simulink model "new_inkine_2020"  (R2022b)
settings: Solver=FixedStepAuto  StartTime=0.0  StopTime=250  FixedStep=0.001  RelTol=1e-3
PreLoadFcn:
  | parameters_new;
InitFcn:
  | parameters_new;
(part 3 of 3)

== matlab function new_inkine_2020/Subsystem/MATLAB Function1 ==
  data: tau0 output; a input; tau output; q input; dq input; d2q input; Wn input; Z2 input; adaptive_rate output
function [tau0,tau,adaptive_rate] = fcn(a,q,dq,d2q, Wn,Z2)
% S1,L1,L3,M1,M2,R2,R1,Le,K1,...
% L2,L11,S3,S4,Lc14,Lc14y,LC1,LC1y,LC2,LC2y,LC3,...
% L9,Lcx10,Ls5,Ls6,Ls11,Ls13,... %杆长与偏置
% I1,I2,I3,I4,I5,I6,I7,I8,I9,I10,I11,I12,I13,I14,I15,...
g=9806.65;theta6=5*pi/6; theta7=-pi/6;
coder.extrinsic('evalin');
L1=0;L3=0;S1=0;R1=0;R2=0;Le=0;K1=0;K2=0;M1=0;M2=0;
L1=evalin('base','L1');L3=evalin('base','L3');S1=evalin('base','S1');R1=evalin('base','R1');Le=evalin('base','Le');R2=evalin('base','R2');
K1=evalin('base','K1');K2=evalin('base','K2');M1=evalin('base','M1');M2=evalin('base','M2');
S1=82;L1=600;L3=550;M1=312.5;M2=140.5;R2=318;
R1=200;Le=414;K1=270;L2=215;L11=532;S3=150;S4=180;
Lc14=100.63;Lc14y=49.13;LC1=192.36;
LC1y=7.69;LC2=-38.71;LC2y=-48.68;LC3=167.99;
L9=sqrt(4.13^2+2.45^2);Lcx10=-13.9;
Ls5=268.5;Ls6=-242.5;Ls11=189; Ls13=189; %偏置

% m1=31.235;m2=17.983;m3=21.85;m4=5.16;m5=2.248;m6=2.248;m7=1.73;m8=1.73;
% m9=121.413;m10=13.425;m11=3.54;m12=1.729;m13=2.99;m14=5.342;m15=2.79;
% I1=[531432.895,1962865.034,1545286.115];
% I2=[118284.16,456199.27,500258.95];
% I3=[79013.25, 1135425.11, 1121439.73];
% I4=[870.60,179377.20,179369.49];
% I5=[3169.766,5265.289,3886.288];%滑块1
% I6=[3169.766,5265.289,3886.288];%滑块2
% I7=[143.00,29009.62,29008.38];
% I8=[143.00,29009.62,29008.38];%AC,BC
% I9=[5187204.097,6638143.629, 4645540.195];
% I10=[230616.784, 122346.017, 246696.850];
% I11=[10700.52,125437.80,115850.13];
% I12=[12209.748,498.623,12408.157];
% I13=[397.49,124363.03,124495.89];
% I14=[18845.358,28753.446,45020.107];
% I15=[376.19,99421.54,99541.62];

m1=51.81;m2=19.166;m3=39.652;m4=8.609;m5=2.248;m6=2.248;m7=3.094;m8=3.094;m9=121.413;m10=11.03; 
m11=8.433;m12=2.164;m13=3.27;m14=5.342;m15=3.585;
I1=[799946.49,3888376.65,3292839.24];
I2=[141847.10, 540821.180,573215.730];
I3=[184132.217, 2737294.136, 2737294.136];
I4=[3478.492,396735.669,396757.714];
I5=[3169.766,5265.289,3886.288];
I6=[3169.766,5265.289,3886.288];
I7=[1032.344, 86107.112,86524.495];
I8=[1032.344, 86107.112,86524.495];
I9=[5187204.097,6638143.629, 4645540.195];
I10=[ 96918.57, 207811.09,  196352.11];
I11=[19267.104,306573.070,298677.886];
I12=[12641.763,1276.684,12641.763];
I13=[1031.019,155951.918, 156712.730];
I14=[18845.358,28753.446,45020.107];
I15=[1180.720,164711.775,165542.954];

K2=K1;L7=Le;L8=L7;Lc11=45+0.5*L11;Lc13=0.5*L1;Lc15=0.5*L3;
% m1=m(1);m2=m(2);m3=m(3);m4=m(4);m5=m(5);m6=m(6);m7=m(7);m8=m(8);m9=m(9);m10=m(10);m11=m(11);m12=m(12);m13=m(13);m14=m(14);m15=m(15);

mload=50;

Ixx1=I1(1); Iyy1=I1(2); Izz1=I1(3);
Ixx2=I2(1); Iyy2=I2(2); Izz2=I2(3);
Ixx3=I3(1); Iyy3=I3(2); Izz3=I3(3);
Ixx4=I4(1); Iyy4=I4(2); Izz4=I4(3);
Ixx5=I5(1); Iyy5=I5(2); Izz5=I5(3);
Ixx6=I6(1); Iyy6=I6(2); Izz6=I6(3);
Ixx7=I7(1); Iyy7=I7(2); Izz7=I7(3);
Ixx8=I8(1); Iyy8=I8(2); Izz8=I8(3);
Ixx9=I9(1); Iyy9=I9(2); Izz9=I9(3);
Ixx10=I10(1);Iyy10=I10(2);Izz10=I10(3);
Ixx11=I11(1);Iyy11=I11(2);Izz11=I11(3);
Ixx12=I12(1);Iyy12=I12(2);Izz12=I12(3);
Ixx13=I13(1);Iyy13=I13(2);Izz13=I13(3);
Ixx14=I14(1);Iyy14=I14(2);Izz14=I14(3);
Ixx15=I15(1);Iyy15=I15(2);Izz15=I15(3);



theta1=q(1);theta4=q(2);theta5=q(3);
theta2=theta6-theta4;theta3=theta7-theta5;
dq1=dq(1);dq2=dq(2);dq3=dq(3);

n=sqrt((M1 - R2*cos(theta3))^2 + (M2 - R2*sin(theta3))^2);n1=1/n;
phi1=asin((K1-R1*sin(theta2))/L7);
phi2=acos((K2-R1*cos(theta2))/L8);
cph1=(L7^2-(K1-R1*sin(theta2))^2)^0.5/L7;

jij9=[ Izz9, 0, 0;0,0,0;0,0,0];Ekr9=0.5*dq.'*jij9*dq;
jmj9=[ L9^2*m9, 0, 0; 0, 0, 0;0, 0, 0];Ekt9=0.5*dq.'*jmj9*dq;

Mm=[Ixx5 + Iyy14/2 + Izz6 + Izz9 + Izz10 + (2*Lc11*m11*sin(theta1)*(M1 - R2*cos(theta5 - theta7))*(Ls11*cos(theta1) - sin(theta1)*(M1 - S1)) - 2*Lc11*m11*cos(theta1)*(M1 - R2*cos(theta5 - theta7))*(Ls11*sin(theta1) + cos(theta1)*(M1 - S1)))*n1 + (Lc11^2*m11*cos(theta1)^2*(M1 - R2*cos(theta5 - theta7))^2 + Lc11^2*m11*sin(theta1)^2*(M1 - R2*cos(theta5 - theta7))^2)*n1^2 + Ixx14/2 - Ixx8*((K2 - R1*cos(theta4 - theta6))^2/L8^2 - 1) + Iyy1*cos(theta4)^2 + Iyy2*cos(theta5)^2 + Iyy3*cos(theta5)^2 + Iyy4*cos(theta4)^2 + Iyy13*cos(theta4)^2 + Iyy15*cos(theta5)^2 - Iyy7*((K1 + R1*sin(theta4 - theta6))^2/L7^2 - 1) + Ixx1*sin(theta4)^2 + Ixx2*sin(theta5)^2 + Ixx3*sin(theta5)^2 + Ixx4*sin(theta4)^2 + Ixx13*sin(theta4)^2 + Ixx15*sin(theta5)^2 + (Iyy8*(K2 - R1*cos(theta4 - theta6))^2)/L8^2 + (Ixx7*(K1 + R1*sin(theta4 - theta6))^2)/L7^2 + Iyy11*n1^2*(M1 - R2*cos(theta5 - theta7))^2 + Ixx11*n1^2*(M2 + R2*sin(theta5 - theta7))^2 + (Ixx12*(M1 - R2*cos(theta5 - theta7))^2)/((M1 - R2*cos(theta5 - theta7))^2 + (M2 + R2*sin(theta5 - theta7))^2) + (Izz12*(M2 + R2*sin(theta5 - theta7))^2)/((M1 - R2*cos(theta5 - theta7))^2 + (M2 + R2*sin(theta5 - theta7))^2) + (m13*(4*Lc13^2*cos(theta4)^2 - 8*Lc13*S1*cos(theta4) - 4*sqrt((3))*Lc13*S3*cos(theta4) + 4*Ls13^2 + 4*S1^2 + 4*sqrt((3))*S1*S3 + 3*S3^2))/4 + m15*(sin(theta1)*(S1 + (sqrt((2))*S4)/2 - L1*cos(theta4) - Lc15*cos(theta5)) + Ls13*cos(theta1))^2 + m15*(cos(theta1)*(S1 + (sqrt((2))*S4)/2 - L1*cos(theta4) - Lc15*cos(theta5)) - Ls13*sin(theta1))^2 + m6*(K2^2 - 2*K2*S1 + Ls6^2 + S1^2) + (m4*(2*S1 - L1*cos(theta4) + 2*L2*cos(theta5))^2)/4 + m3*(L1*cos(theta4) - S1 + LC3*cos(theta5))^2 + m1*(LC1*cos(theta4) - S1 + LC1y*sin(theta4))^2 + (m14*(cos(theta1)*(Lc14y + 2*S1 - sqrt((3))*Lc14 + sqrt((3))*S3 - 2*L1*cos(theta4)) - 2*Ls13*sin(theta1))^2)/4 + (m14*(sin(theta1)*(Lc14y + 2*S1 - sqrt((3))*Lc14 + sqrt((3))*S3 - 2*L1*cos(theta4)) + 2*Ls13*cos(theta1))^2)/4 + m10*(Lcx10 - S1 + L1*cos(theta4) + L3*cos(theta5))^2 + m5*(sin(theta1)*(S1 + sqrt(L7^2 - (K1 + R1*sin(theta4 - theta6))^2) - R1*cos(theta4 - theta6)) + Ls5*cos(theta1))^2 + m5*(cos(theta1)*(S1 + sqrt(L7^2 - (K1 + R1*sin(theta4 - theta6))^2) - R1*cos(theta4 - theta6)) - Ls5*sin(theta1))^2 + (m7*(L7^2*cph1^2 - 4*L7*R1*cph1*cos(theta4 - theta6) + 4*L7*S1*cph1 + 4*Ls5^2 + 4*R1^2*cos(theta4 - theta6)^2 - 8*R1*S1*cos(theta4 - theta6) + 4*S1^2))/4 + L9^2*m9 + (m8*(K2^2 + 2*K2*R1*cos(theta4 - theta6) - 4*K2*S1 + 4*Ls6^2 + R1^2*cos(theta4 - theta6)^2 - 4*R1*S1*cos(theta4 - theta6) + 4*S1^2))/4 + m12*(S1 - R2*cos(theta5 - theta7))^2 + m11*(Ls11*sin(theta1) + cos(theta1)*(M1 - S1))^2 + m11*(Ls11*cos(theta1) - sin(theta1)*(M1 - S1))^2 + m2*(S1 + LC2*cos(theta5) - LC2y*sin(theta5))^2, - L1*Ls13*m14*sin(theta4) - L1*Ls13*m15*sin(theta4) - Lc13*Ls13*m13*sin(theta4) - (Ls6*R1*m8*sin(theta4 - theta6))/2 + (Ls5*R1*m5*((R1*sin(2*theta4 - 2*theta6))/2 - sin(theta4 - theta6)*sqrt(L7^2 - (K1 + R1*sin(theta4 - theta6))^2) + K1*cos(theta4 - theta6)))/sqrt(L7^2 - (K1 + R1*sin(theta4 - theta6))^2) + (Ls5*R1*m7*(K1*cos(theta4 - theta6) - 2*L7*cph1*sin(theta4 - theta6) + R1*cos(theta4 - theta6)*sin(theta4 - theta6)))/(2*L7*cph1), (-Lc11*Ls11*R2*m11*(M2 + R2*sin(theta5 - theta7))*(R2 - M1*cos(theta5 - theta7) + M2*sin(theta5 - theta7)))*n1^3 - Lc15*Ls13*m15*sin(theta5); - L1*Ls13*m14*sin(theta4) - L1*Ls13*m15*sin(theta4) - Lc13*Ls13*m13*sin(theta4) - (Ls6*R1*m8*sin(theta4 - theta6))/2 + (Ls5*R1*m5*((R1*sin(2*theta4 - 2*theta6))/2 - sin(theta4 - theta6)*sqrt(L7^2 - (K1 + R1*sin(theta4 - theta6))^2) + K1*cos(theta4 - theta6)))/sqrt(L7^2 - (K1 + R1*sin(theta4 - theta6))^2) + (Ls5*R1*m7*(K1*cos(theta4 - theta6) - 2*L7*cph1*sin(theta4 - theta6) + R1*cos(theta4 - theta6)*sin(theta4 - theta6)))/(2*L7*cph1), Izz1 + Izz4 + Izz13 + m6*(R1*cos(theta4 - theta6) - (R1*sin(theta4 - theta6)*(K2 - R1*cos(theta4 - theta6)))/sqrt(L7^2 - (K2 - R1*cos(theta4 - theta6))^2))^2 + L1^2*m10 + L1^2*m3 + (L1^2*m4)/4 + L1^2*m14 + L1^2*m15 + Lc13^2*m13 + m1*(LC1^2 + LC1y^2) + m8*(R1*cos(theta4 - theta6) - (R1*sin(theta4 - theta6)*(K2 - R1*cos(theta4 - theta6)))/(L8*sqrt(1 - (K2 - R1*cos(theta4 - theta6))^2/L8^2)*2))^2 + m7*cos(theta1)^2*(R1*sin(theta4 - theta6) - (R1*cos(theta4 - theta6)*(K1 + R1*sin(theta4 - theta6)))/(2*L7*cph1))^2 + m7*sin(theta1)^2*(R1*sin(theta4 - theta6) - (R1*cos(theta4 - theta6)*(K1 + R1*sin(theta4 - theta6)))/(2*L7*cph1))^2 + m5*cos(theta1)^2*(R1*sin(theta4 - theta6) - (R1*cos(theta4 - theta6)*(K1 + R1*sin(theta4 - theta6)))/sqrt(L7^2 - (K1 + R1*sin(theta4 - theta6))^2))^2 + m5*sin(theta1)^2*(R1*sin(theta4 - theta6) - (R1*cos(theta4 - theta6)*(K1 + R1*sin(theta4 - theta6)))/sqrt(L7^2 - (K1 + R1*sin(theta4 - theta6))^2))^2 + (R1^2*m7*cos(theta4 - theta6)^2)/4 + (R1^2*m8*sin(theta4 - theta6)^2*cos(theta1)^2)/4 + (R1^2*m8*sin(theta4 - theta6)^2*sin(theta1)^2)/4 - (Izz7*R1^2*cos(theta4 - theta6)^2)/(L7^2*((K1 + R1*sin(theta4 - theta6))^2/L7^2 - 1)) - (Izz8*R1^2*sin(theta4 - theta6)^2)/(L8^2*((K2 - R1*cos(theta4 - theta6))^2/L8^2 - 1)), L1*L3*cos(theta4 - theta5)*m10 - (L1*L2*m4*cos(theta4 - theta5))/2 + L1*LC3*m3*cos(theta4 - theta5) + L1*Lc15*m15*cos(theta4 - theta5); (-Lc11*Ls11*R2*m11*(M2 + R2*sin(theta5 - theta7))*(R2 - M1*cos(theta5 - theta7) + M2*sin(theta5 - theta7)))*n1^3 - Lc15*Ls13*m15*sin(theta5), L1*L3*cos(theta4 - theta5)*m10 - (L1*L2*m4*cos(theta4 - theta5))/2 + L1*LC3*m3*cos(theta4 - theta5) + L1*Lc15*m15*cos(theta4 - theta5), Izz2 + Izz3 + Izz15 + (Lc11^2*R2^2*m11*(M1 - R2*cos(theta5 - theta7))^2*(R2 - M1*cos(theta5 - theta7) + M2*sin(theta5 - theta7))^2 + Lc11^2*R2^2*m11*cos(theta1)^2*(M2 + R2*sin(theta5 - theta7))^2*(R2 - M1*cos(theta5 - theta7) + M2*sin(theta5 - theta7))^2 + Lc11^2*R2^2*m11*sin(theta1)^2*(M2 + R2*sin(theta5 - theta7))^2*(R2 - M1*cos(theta5 - theta7) + M2*sin(theta5 - theta7))^2)*n1^6 - (Iyy12*((R2*sin(theta5 - theta7))/sqrt(((M1 - R2*cos(theta5 - theta7))^2 + (M2 + R2*sin(theta5 - theta7))^2)) - ((M1 - R2*cos(theta5 - theta7))*(2*R2*cos(theta5 - theta7)*(M2 + R2*sin(theta5 - theta7)) + 2*R2*sin(theta5 - theta7)*(M1 - R2*cos(theta5 - theta7))))/(2*((M1 - R2*cos(theta5 - theta7))^2 + (M2 + R2*sin(theta5 - theta7))^2)^(3/2)))^2)/((M1 - R2*cos(theta5 - theta7))^2/((M1 - R2*cos(theta5 - theta7))^2 + (M2 + R2*sin(theta5 - theta7))^2) - 1) + Izz11*R2^2*n1^4*(R2 - M1*cos(theta5 - theta7) + M2*sin(theta5 - theta7))^2 + m4*L2^2 + m10*L3^2 + m3*LC3^2 + m15*Lc15^2 + m12*R2^2 + m2*(LC2^2 + LC2y^2)];

V2=[dq1*((dq3*(2*R2*m11*sin(theta5 - theta7)*(M1 - R2*cos(theta5 - theta7))*Lc11^2*cos(theta1)^2 + 2*R2*m11*sin(theta5 - theta7)*(M1 - R2*cos(theta5 - theta7))*Lc11^2*sin(theta1)^2)*n1^2)/2 - (dq3*(2*Lc11*R2*m11*sin(theta5 - theta7)*cos(theta1)*(Ls11*sin(theta1) + cos(theta1)*(M1 - S1)) - 2*Lc11*R2*m11*sin(theta5 - theta7)*sin(theta1)*(Ls11*cos(theta1) - sin(theta1)*(M1 - S1)))*n1)/2 + (dq2*((m13*(8*Lc13*S1*sin(theta4) - 8*Lc13^2*cos(theta4)*sin(theta4) + 4*sqrt((3))*Lc13*S3*sin(theta4)))/4 - (m8*(2*K2*R1*sin(theta4 - theta6) - 4*R1*S1*sin(theta4 - theta6) + 2*R1^2*cos(theta4 - theta6)*sin(theta4 - theta6)))/4 + (m7*(8*R1*S1*sin(theta4 - theta6) - 8*R1^2*cos(theta4 - theta6)*sin(theta4 - theta6) + 4*L7*R1*cph1*sin(theta4 - theta6)))/4 + 2*Ixx1*cos(theta4)*sin(theta4) + 2*Ixx4*cos(theta4)*sin(theta4) + 2*Ixx13*cos(theta4)*sin(theta4) - 2*Iyy1*cos(theta4)*sin(theta4) - 2*Iyy4*cos(theta4)*sin(theta4) - 2*Iyy13*cos(theta4)*sin(theta4) + 2*m1*(LC1y*cos(theta4) - LC1*sin(theta4))*(LC1*cos(theta4) - S1 + LC1y*sin(theta4)) + (L1*m4*sin(theta4)*(2*S1 - L1*cos(theta4) + 2*L2*cos(theta5)))/2 - 2*L1*m3*sin(theta4)*(L1*cos(theta4) - S1 + LC3*cos(theta5)) - 2*L1*sin(theta4)*m10*(Lcx10 - S1 + L1*cos(theta4) + L3*cos(theta5)) + 2*m5*cos(theta1)*(cos(theta1)*(S1 + sqrt((L7^2 - (K1 + R1*sin(theta4 - theta6))^2)) - R1*cos(theta4 - theta6)) - Ls5*sin(theta1))*(R1*sin(theta4 - theta6) - (R1*cos(theta4 - theta6)*(K1 + R1*sin(theta4 - theta6)))/sqrt(L7^2 - (K1 + R1*sin(theta4 - theta6))^2)) + 2*m5*sin(theta1)*(sin(theta1)*(S1 + sqrt((L7^2 - (K1 + R1*sin(theta4 - theta6))^2)) - R1*cos(theta4 - theta6)) + Ls5*cos(theta1))*(R1*sin(theta4 - theta6) - (R1*cos(theta4 - theta6)*(K1 + R1*sin(theta4 - theta6)))/sqrt(L7^2 - (K1 + R1*sin(theta4 - theta6))^2)) + L1*m14*cos(theta1)*sin(theta4)*(cos(theta1)*(Lc14y + 2*S1 - sqrt((3))*Lc14 + sqrt((3))*S3 - 2*L1*cos(theta4)) - 2*Ls13*sin(theta1)) + L1*m14*sin(theta1)*sin(theta4)*(sin(theta1)*(Lc14y + 2*S1 - sqrt((3))*Lc14 + sqrt((3))*S3 - 2*L1*cos(theta4)) + 2*Ls13*cos(theta1)) + (2*Ixx7*R1*cos(theta4 - theta6)*(K1 + R1*sin(theta4 - theta6)))/L7^2 - (2*Ixx8*R1*sin(theta4 - theta6)*(K2 - R1*cos(theta4 - theta6)))/L8^2 - (2*Iyy7*R1*cos(theta4 - theta6)*(K1 + R1*sin(theta4 - theta6)))/L7^2 + (2*Iyy8*R1*sin(theta4 - theta6)*(K2 - R1*cos(theta4 - theta6)))/L8^2 + 2*L1*m15*cos(theta1)*sin(theta4)*(cos(theta1)*(S1 + (sqrt((2))*S4)/2 - L1*cos(theta4) - Lc15*cos(theta5)) - Ls13*sin(theta1)) + 2*L1*m15*sin(theta1)*sin(theta4)*(sin(theta1)*(S1 + (sqrt((2))*S4)/2 - L1*cos(theta4) - Lc15*cos(theta5)) + Ls13*cos(theta1))))/2 + (dq3*(2*Ixx2*cos(theta5)*sin(theta5) - 2*m2*(LC2y*cos(theta5) + LC2*sin(theta5))*(S1 + LC2*cos(theta5) - LC2y*sin(theta5)) + 2*Ixx3*cos(theta5)*sin(theta5) + 2*Ixx15*cos(theta5)*sin(theta5) - 2*Iyy2*cos(theta5)*sin(theta5) - 2*Iyy3*cos(theta5)*sin(theta5) - 2*Iyy15*cos(theta5)*sin(theta5) - L2*m4*sin(theta5)*(2*S1 - L1*cos(theta4) + 2*L2*cos(theta5)) - 2*LC3*m3*sin(theta5)*(L1*cos(theta4) - S1 + LC3*cos(theta5)) - 2*L3*sin(theta5)*m10*(Lcx10 - S1 + L1*cos(theta4) + L3*cos(theta5)) - (Ixx12*(M1 - R2*cos(theta5 - theta7))^2*(2*R2*cos(theta5 - theta7)*(M2 + R2*sin(theta5 - theta7)) + 2*R2*sin(theta5 - theta7)*(M1 - R2*cos(theta5 - theta7))))/((M1 - R2*cos(theta5 - theta7))^2 + (M2 + R2*sin(theta5 - theta7))^2)^2 + 2*R2*m12*sin(theta5 - theta7)*(S1 - R2*cos(theta5 - theta7)) - (Izz12*(M2 + R2*sin(theta5 - theta7))^2*(2*R2*cos(theta5 - theta7)*(M2 + R2*sin(theta5 - theta7)) + 2*R2*sin(theta5 - theta7)*(M1 - R2*cos(theta5 - theta7))))/((M1 - R2*cos(theta5 - theta7))^2 + (M2 + R2*sin(theta5 - theta7))^2)^2 + 2*Ixx11*R2*n1^2*cos(theta5 - theta7)*(M2 + R2*sin(theta5 - theta7)) + 2*Iyy11*R2*n1^2*sin(theta5 - theta7)*(M1 - R2*cos(theta5 - theta7)) + 2*Lc15*m15*cos(theta1)*sin(theta5)*(cos(theta1)*(S1 + (sqrt((2))*S4)/2 - L1*cos(theta4) - Lc15*cos(theta5)) - Ls13*sin(theta1)) + 2*Lc15*m15*sin(theta1)*sin(theta5)*(sin(theta1)*(S1 + (sqrt((2))*S4)/2 - L1*cos(theta4) - Lc15*cos(theta5)) + Ls13*cos(theta1)) + (2*Ixx12*R2*sin(theta5 - theta7)*(M1 - R2*cos(theta5 - theta7)))/((M1 - R2*cos(theta5 - theta7))^2 + (M2 + R2*sin(theta5 - theta7))^2) + (2*Izz12*R2*cos(theta5 - theta7)*(M2 + R2*sin(theta5 - theta7)))/((M1 - R2*cos(theta5 - theta7))^2 + (M2 + R2*sin(theta5 - theta7))^2)))/2) - dq2*(dq2*(L1*Ls13*m14*cos(theta4) + L1*Ls13*m15*cos(theta4) + Lc13*Ls13*m13*cos(theta4) + (Ls6*R1*m8*cos(theta4 - theta6))/2 + (Ls5*R1*m5*(cos(theta4 - theta6)*sqrt((L7^2 - (K1 + R1*sin(theta4 - theta6))^2)) - R1*cos(2*theta4 - 2*theta6) + K1*sin(theta4 - theta6) - (R1*cos(theta4 - theta6)*sin(theta4 - theta6)*(K1 + R1*sin(theta4 - theta6)))/sqrt((L7^2 - (K1 + R1*sin(theta4 - theta6))^2))))/sqrt((L7^2 - (K1 + R1*sin(theta4 - theta6))^2)) + (Ls5*R1*m7*(- R1*cos(theta4 - theta6)^2 + 2*L7*cph1*cos(theta4 - theta6) + R1*sin(theta4 - theta6)^2 + K1*sin(theta4 - theta6)))/(2*L7*cph1) - (Ls5*R1^2*m5*cos(theta4 - theta6)*(K1 + R1*sin(theta4 - theta6))*((R1*sin(2*theta4 - 2*theta6))/2 - sin(theta4 - theta6)*sqrt((L7^2 - (K1 + R1*sin(theta4 - theta6))^2)) + K1*cos(theta4 - theta6)))/(L7^2 - (K1 + R1*sin(theta4 - theta6))^2)^(3/2)) - (dq1*((m13*(8*Lc13*S1*sin(theta4) - 8*Lc13^2*cos(theta4)*sin(theta4) + 4*sqrt((3))*Lc13*S3*sin(theta4)))/4 - (m8*(2*K2*R1*sin(theta4 - theta6) - 4*R1*S1*sin(theta4 - theta6) + 2*R1^2*cos(theta4 - theta6)*sin(theta4 - theta6)))/4 + (m7*(8*R1*S1*sin(theta4 - theta6) - 8*R1^2*cos(theta4 - theta6)*sin(theta4 - theta6) + 4*L7*R1*cph1*sin(theta4 - theta6)))/4 + 2*Ixx1*cos(theta4)*sin(theta4) + 2*Ixx4*cos(theta4)*sin(theta4) + 2*Ixx13*cos(theta4)*sin(theta4) - 2*Iyy1*cos(theta4)*sin(theta4) - 2*Iyy4*cos(theta4)*sin(theta4) - 2*Iyy13*cos(theta4)*sin(theta4) + 2*m1*(LC1y*cos(theta4) - LC1*sin(theta4))*(LC1*cos(theta4) - S1 + LC1y*sin(theta4)) + (L1*m4*sin(theta4)*(2*S1 - L1*cos(theta4) + 2*L2*cos(theta5)))/2 - 2*L1*m3*sin(theta4)*(L1*cos(theta4) - S1 + LC3*cos(theta5)) - 2*L1*sin(theta4)*m10*(Lcx10 - S1 + L1*cos(theta4) + L3*cos(theta5)) + 2*m5*cos(theta1)*(cos(theta1)*(S1 + sqrt((L7^2 - (K1 + R1*sin(theta4 - theta6))^2)) - R1*cos(theta4 - theta6)) - Ls5*sin(theta1))*(R1*sin(theta4 - theta6) - (R1*cos(theta4 - theta6)*(K1 + R1*sin(theta4 - theta6)))/sqrt(L7^2 - (K1 + R1*sin(theta4 - theta6))^2)) + 2*m5*sin(theta1)*(sin(theta1)*(S1 + sqrt((L7^2 - (K1 + R1*sin(theta4 - theta6))^2)) - R1*cos(theta4 - theta6)) + Ls5*cos(theta1))*(R1*sin(theta4 - theta6) - (R1*cos(theta4 - theta6)*(K1 + R1*sin(theta4 - theta6)))/sqrt(L7^2 - (K1 + R1*sin(theta4 - theta6))^2)) + L1*m14*cos(theta1)*sin(theta4)*(cos(theta1)*(Lc14y + 2*S1 - sqrt((3))*Lc14 + sqrt((3))*S3 - 2*L1*cos(theta4)) - 2*Ls13*sin(theta1)) + L1*m14*sin(theta1)*sin(theta4)*(sin(theta1)*(Lc14y + 2*S1 - sqrt((3))*Lc14 + sqrt((3))*S3 - 2*L1*cos(theta4)) + 2*Ls13*cos(theta1)) + (2*Ixx7*R1*cos(theta4 - theta6)*(K1 + R1*sin(theta4 - theta6)))/L7^2 - (2*Ixx8*R1*sin(theta4 - theta6)*(K2 - R1*cos(theta4 - theta6)))/L8^2 - (2*Iyy7*R1*cos(theta4 - theta6)*(K1 + R1*sin(theta4 - theta6)))/L7^2 + (2*Iyy8*R1*sin(theta4 - theta6)*(K2 - R1*cos(theta4 - theta6)))/L8^2 + 2*L1*m15*cos(theta1)*sin(theta4)*(cos(theta1)*(S1 + (sqrt((2))*S4)/2 - L1*cos(theta4) - Lc15*cos(theta5)) - Ls13*sin(theta1)) + 2*L1*m15*sin(theta1)*sin(theta4)*(sin(theta1)*(S1 + (sqrt((2))*S4)/2 - L1*cos(theta4) - Lc15*cos(theta5)) + Ls13*cos(theta1))))/2) - dq3*((dq3*((Lc11*Ls11*R2*m11*(M2 + R2*sin(theta5 - theta7))*(M2*cos(theta5 - theta7) + M1*sin(theta5 - theta7)) + Lc11*Ls11*R2^2*m11*cos(theta5 - theta7)*(R2 - M1*cos(theta5 - theta7) + M2*sin(theta5 - theta7)))*n1^3 + Lc15*Ls13*m15*cos(theta5)))/2 - (dq1*(n1^2*(2*R2*m11*sin(theta5 - theta7)*(M1 - R2*cos(theta5 - theta7))*Lc11^2*cos(theta1)^2 + 2*R2*m11*sin(theta5 - theta7)*(M1 - R2*cos(theta5 - theta7))*Lc11^2*sin(theta1)^2) - n1*(2*Lc11*R2*m11*sin(theta5 - theta7)*cos(theta1)*(Ls11*sin(theta1) + cos(theta1)*(M1 - S1)) - 2*Lc11*R2*m11*sin(theta5 - theta7)*sin(theta1)*(Ls11*cos(theta1) - sin(theta1)*(M1 - S1))) - 2*m2*(LC2y*cos(theta5) + LC2*sin(theta5))*(S1 + LC2*cos(theta5) - LC2y*sin(theta5)) + 2*Ixx2*cos(theta5)*sin(theta5) + 2*Ixx3*cos(theta5)*sin(theta5) + 2*Ixx15*cos(theta5)*sin(theta5) - 2*Iyy2*cos(theta5)*sin(theta5) - 2*Iyy3*cos(theta5)*sin(theta5) - 2*Iyy15*cos(theta5)*sin(theta5) - L2*m4*sin(theta5)*(2*S1 - L1*cos(theta4) + 2*L2*cos(theta5)) - 2*LC3*m3*sin(theta5)*(L1*cos(theta4) - S1 + LC3*cos(theta5)) - 2*L3*sin(theta5)*m10*(Lcx10 - S1 + L1*cos(theta4) + L3*cos(theta5)) - (Ixx12*(M1 - R2*cos(theta5 - theta7))^2*(2*R2*cos(theta5 - theta7)*(M2 + R2*sin(theta5 - theta7)) + 2*R2*sin(theta5 - theta7)*(M1 - R2*cos(theta5 - theta7))))/((M1 - R2*cos(theta5 - theta7))^2 + (M2 + R2*sin(theta5 - theta7))^2)^2 + 2*R2*m12*sin(theta5 - theta7)*(S1 - R2*cos(theta5 - theta7)) - (Izz12*(M2 + R2*sin(theta5 - theta7))^2*(2*R2*cos(theta5 - theta7)*(M2 + R2*sin(theta5 - theta7)) + 2*R2*sin(theta5 - theta7)*(M1 - R2*cos(theta5 - theta7))))/((M1 - R2*cos(theta5 - theta7))^2 + (M2 + R2*sin(theta5 - theta7))^2)^2 + 2*Ixx11*R2*n1^2*cos(theta5 - theta7)*(M2 + R2*sin(theta5 - theta7)) + 2*Iyy11*R2*n1^2*sin(theta5 - theta7)*(M1 - R2*cos(theta5 - theta7)) + 2*Lc15*m15*cos(theta1)*sin(theta5)*(cos(theta1)*(S1 + (sqrt((2))*S4)/2 - L1*cos(theta4) - Lc15*cos(theta5)) - Ls13*sin(theta1)) + 2*Lc15*m15*sin(theta1)*sin(theta5)*(sin(theta1)*(S1 + (sqrt((2))*S4)/2 - L1*cos(theta4) - Lc15*cos(theta5)) + Ls13*cos(theta1)) + (2*Ixx12*R2*sin(theta5 - theta7)*(M1 - R2*cos(theta5 - theta7)))/((M1 - R2*cos(theta5 - theta7))^2 + (M2 + R2*sin(theta5 - theta7))^2) + (2*Izz12*R2*cos(theta5 - theta7)*(M2 + R2*sin(theta5 - theta7)))/((M1 - R2*cos(theta5 - theta7))^2 + (M2 + R2*sin(theta5 - theta7))^2)))/2 + (dq3*n1^3*(Lc11*Ls11*R2*m11*(M2 + R2*sin(theta5 - theta7))*(M2*cos(theta5 - theta7) + M1*sin(theta5 - theta7)) + Lc11*Ls11*R2^2*m11*cos(theta5 - theta7)*(R2 - M1*cos(theta5 - theta7) + M2*sin(theta5 - theta7))))/2 + (Lc15*Ls13*dq3*m15*cos(theta5))/2); dq3^2*(L1*L3*sin(theta4 - theta5)*m10 - (L1*L2*m4*sin(theta4 - theta5))/2 + L1*LC3*m3*sin(theta4 - theta5) + L1*Lc15*m15*sin(theta4 - theta5)) + (dq2^2*(2*m5*cos(theta1)^2*(R1*sin(theta4 - theta6) - (R1*cos(theta4 - theta6)*(K1 + R1*sin(theta4 - theta6)))/sqrt(L7^2 - (K1 + R1*sin(theta4 - theta6))^2))*(R1*cos(theta4 - theta6) - (R1^2*cos(theta4 - theta6)^2)/sqrt(L7^2 - (K1 + R1*sin(theta4 - theta6))^2) + (R1*sin(theta4 - theta6)*(K1 + R1*sin(theta4 - theta6)))/sqrt(L7^2 - (K1 + R1*sin(theta4 - theta6))^2) - (R1^2*cos(theta4 - theta6)^2*(K1 + R1*sin(theta4 - theta6))^2)/(L7^2 - (K1 + R1*sin(theta4 - theta6))^2)^(3/2)) - 2*m6*(R1*cos(theta4 - theta6) - (R1*sin(theta4 - theta6)*(K2 - R1*cos(theta4 - theta6)))/sqrt(L7^2 - (K2 - R1*cos(theta4 - theta6))^2))*(R1*sin(theta4 - theta6) + (R1^2*sin(theta4 - theta6)^2)/sqrt(L7^2 - (K2 - R1*cos(theta4 - theta6))^2) + (R1*cos(theta4 - theta6)*(K2 - R1*cos(theta4 - theta6)))/sqrt(L7^2 - (K2 - R1*cos(theta4 - theta6))^2) + (R1^2*sin(theta4 - theta6)^2*(K2 - R1*cos(theta4 - theta6))^2)/(L7^2 - (K2 - R1*cos(theta4 - theta6))^2)^(3/2)) - 2*m8*(R1*cos(theta4 - theta6) - (R1*sin(theta4 - theta6)*(K2 - R1*cos(theta4 - theta6)))/(2*L8*sqrt(1 - (K2 - R1*cos(theta4 - theta6))^2/L8^2)))*(R1*sin(theta4 - theta6) + (R1^2*sin(theta4 - theta6)^2)/(2*L8*sqrt(1 - (K2 - R1*cos(theta4 - theta6))^2/L8^2)) + (R1*cos(theta4 - theta6)*(K2 - R1*cos(theta4 - theta6)))/(2*L8*sqrt(1 - (K2 - R1*cos(theta4 - theta6))^2/L8^2)) + (R1^2*sin(theta4 - theta6)^2*(K2 - R1*cos(theta4 - theta6))^2)/(2*L8^3*(1 - (K2 - R1*cos(theta4 - theta6))^2/L8^2)^(3/2))) + 2*m5*sin(theta1)^2*(R1*sin(theta4 - theta6) - (R1*cos(theta4 - theta6)*(K1 + R1*sin(theta4 - theta6)))/sqrt(L7^2 - (K1 + R1*sin(theta4 - theta6))^2))*(R1*cos(theta4 - theta6) - (R1^2*cos(theta4 - theta6)^2)/sqrt(L7^2 - (K1 + R1*sin(theta4 - theta6))^2) + (R1*sin(theta4 - theta6)*(K1 + R1*sin(theta4 - theta6)))/sqrt(L7^2 - (K1 + R1*sin(theta4 - theta6))^2) - (R1^2*cos(theta4 - theta6)^2*(K1 + R1*sin(theta4 - theta6))^2)/(L7^2 - (K1 + R1*sin(theta4 - theta6))^2)^(3/2)) + 2*m7*cos(theta1)^2*(R1*sin(theta4 - theta6) - (R1*cos(theta4 - theta6)*(K1 + R1*sin(theta4 - theta6)))/(2*L7*cph1))*(R1*cos(theta4 - theta6) - (R1^2*cos(theta4 - theta6)^2)/(2*L7*cph1) + (R1*sin(theta4 - theta6)*(K1 + R1*sin(theta4 - theta6)))/(2*L7*cph1)) + 2*m7*sin(theta1)^2*(R1*sin(theta4 - theta6) - (R1*cos(theta4 - theta6)*(K1 + R1*sin(theta4 - theta6)))/(2*L7*cph1))*(R1*cos(theta4 - theta6) - (R1^2*cos(theta4 - theta6)^2)/(2*L7*cph1) + (R1*sin(theta4 - theta6)*(K1 + R1*sin(theta4 - theta6)))/(2*L7*cph1)) - (R1^2*m7*cos(theta4 - theta6)*sin(theta4 - theta6))/2 + (R1^2*m8*cos(theta4 - theta6)*sin(theta4 - theta6)*cos(theta1)^2)/2 + (R1^2*m8*cos(theta4 - theta6)*sin(theta4 - theta6)*sin(theta1)^2)/2 + (2*Izz8*R1^3*sin(theta4 - theta6)^3*(K2 - R1*cos(theta4 - theta6)))/(L8^4*((K2 - R1*cos(theta4 - theta6))^2/L8^2 - 1)^2) + (2*Izz7*R1^3*cos(theta4 - theta6)^3*(K1 + R1*sin(theta4 - theta6)))/(L7^4*((K1 + R1*sin(theta4 - theta6))^2/L7^2 - 1)^2) - (2*Izz8*R1^2*cos(theta4 - theta6)*sin(theta4 - theta6))/(L8^2*((K2 - R1*cos(theta4 - theta6))^2/L8^2 - 1)) + (2*Izz7*R1^2*cos(theta4 - theta6)*sin(theta4 - theta6))/(L7^2*((K1 + R1*sin(theta4 - theta6))^2/L7^2 - 1))))/2 - (dq1^2*((m13*(8*Lc13*S1*sin(theta4) - 8*Lc13^2*cos(theta4)*sin(theta4) + 4*sqrt((3))*Lc13*S3*sin(theta4)))/4 - (m8*(2*K2*R1*sin(theta4 - theta6) - 4*R1*S1*sin(theta4 - theta6) + 2*R1^2*cos(theta4 - theta6)*sin(theta4 - theta6)))/4 + (m7*(8*R1*S1*sin(theta4 - theta6) - 8*R1^2*cos(theta4 - theta6)*sin(theta4 - theta6) + 4*L7*R1*cph1*sin(theta4 - theta6)))/4 + 2*Ixx1*cos(theta4)*sin(theta4) + 2*Ixx4*cos(theta4)*sin(theta4) + 2*Ixx13*cos(theta4)*sin(theta4) - 2*Iyy1*cos(theta4)*sin(theta4) - 2*Iyy4*cos(theta4)*sin(theta4) - 2*Iyy13*cos(theta4)*sin(theta4) + 2*m1*(LC1y*cos(theta4) - LC1*sin(theta4))*(LC1*cos(theta4) - S1 + LC1y*sin(theta4)) + (L1*m4*sin(theta4)*(2*S1 - L1*cos(theta4) + 2*L2*cos(theta5)))/2 - 2*L1*m3*sin(theta4)*(L1*cos(theta4) - S1 + LC3*cos(theta5)) - 2*L1*sin(theta4)*m10*(Lcx10 - S1 + L1*cos(theta4) + L3*cos(theta5)) + 2*m5*cos(theta1)*(cos(theta1)*(S1 + sqrt((L7^2 - (K1 + R1*sin(theta4 - theta6))^2)) - R1*cos(theta4 - theta6)) - Ls5*sin(theta1))*(R1*sin(theta4 - theta6) - (R1*cos(theta4 - theta6)*(K1 + R1*sin(theta4 - theta6)))/sqrt(L7^2 - (K1 + R1*sin(theta4 - theta6))^2)) + 2*m5*sin(theta1)*(sin(theta1)*(S1 + sqrt((L7^2 - (K1 + R1*sin(theta4 - theta6))^2)) - R1*cos(theta4 - theta6)) + Ls5*cos(theta1))*(R1*sin(theta4 - theta6) - (R1*cos(theta4 - theta6)*(K1 + R1*sin(theta4 - theta6)))/sqrt(L7^2 - (K1 + R1*sin(theta4 - theta6))^2)) + L1*m14*cos(theta1)*sin(theta4)*(cos(theta1)*(Lc14y + 2*S1 - sqrt((3))*Lc14 + sqrt((3))*S3 - 2*L1*cos(theta4)) - 2*Ls13*sin(theta1)) + L1*m14*sin(theta1)*sin(theta4)*(sin(theta1)*(Lc14y + 2*S1 - sqrt((3))*Lc14 + sqrt((3))*S3 - 2*L1*cos(theta4)) + 2*Ls13*cos(theta1)) + (2*Ixx7*R1*cos(theta4 - theta6)*(K1 + R1*sin(theta4 - theta6)))/L7^2 - (2*Ixx8*R1*sin(theta4 - theta6)*(K2 - R1*cos(theta4 - theta6)))/L8^2 - (2*Iyy7*R1*cos(theta4 - theta6)*(K1 + R1*sin(theta4 - theta6)))/L7^2 + (2*Iyy8*R1*sin(theta4 - theta6)*(K2 - R1*cos(theta4 - theta6)))/L8^2 + 2*L1*m15*cos(theta1)*sin(theta4)*(cos(theta1)*(S1 + (sqrt((2))*S4)/2 - L1*cos(theta4) - Lc15*cos(theta5)) - Ls13*sin(theta1)) + 2*L1*m15*sin(theta1)*sin(theta4)*(sin(theta1)*(S1 + (sqrt((2))*S4)/2 - L1*cos(theta4) - Lc15*cos(theta5)) + Ls13*cos(theta1))))/2; ((L1*L2*m4*sin(theta4 - theta5))/2 - L1*L3*sin(theta4 - theta5)*m10 - L1*LC3*m3*sin(theta4 - theta5) - L1*Lc15*m15*sin(theta4 - theta5))*dq2^2 - dq1*((dq1*(n1^2*(2*R2*m11*sin(theta5 - theta7)*(M1 - R2*cos(theta5 - theta7))*Lc11^2*cos(theta1)^2 + 2*R2*m11*sin(theta5 - theta7)*(M1 - R2*cos(theta5 - theta7))*Lc11^2*sin(theta1)^2) - n1*(2*Lc11*R2*m11*sin(theta5 - theta7)*cos(theta1)*(Ls11*sin(theta1) + cos(theta1)*(M1 - S1)) - 2*Lc11*R2*m11*sin(theta5 - theta7)*sin(theta1)*(Ls11*cos(theta1) - sin(theta1)*(M1 - S1))) - 2*m2*(LC2y*cos(theta5) + LC2*sin(theta5))*(S1 + LC2*cos(theta5) - LC2y*sin(theta5)) + 2*Ixx2*cos(theta5)*sin(theta5) + 2*Ixx3*cos(theta5)*sin(theta5) + 2*Ixx15*cos(theta5)*sin(theta5) - 2*Iyy2*cos(theta5)*sin(theta5) - 2*Iyy3*cos(theta5)*sin(theta5) - 2*Iyy15*cos(theta5)*sin(theta5) - L2*m4*sin(theta5)*(2*S1 - L1*cos(theta4) + 2*L2*cos(theta5)) - 2*LC3*m3*sin(theta5)*(L1*cos(theta4) - S1 + LC3*cos(theta5)) - 2*L3*sin(theta5)*m10*(Lcx10 - S1 + L1*cos(theta4) + L3*cos(theta5)) - (Ixx12*(M1 - R2*cos(theta5 - theta7))^2*(2*R2*cos(theta5 - theta7)*(M2 + R2*sin(theta5 - theta7)) + 2*R2*sin(theta5 - theta7)*(M1 - R2*cos(theta5 - theta7))))/((M1 - R2*cos(theta5 - theta7))^2 + (M2 + R2*sin(theta5 - theta7))^2)^2 + 2*R2*m12*sin(theta5 - theta7)*(S1 - R2*cos(theta5 - theta7)) - (Izz12*(M2 + R2*sin(theta5 - theta7))^2*(2*R2*cos(theta5 - theta7)*(M2 + R2*sin(theta5 - theta7)) + 2*R2*sin(theta5 - theta7)*(M1 - R2*cos(theta5 - theta7))))/((M1 - R2*cos(theta5 - theta7))^2 + (M2 + R2*sin(theta5 - theta7))^2)^2 + 2*Ixx11*R2*n1^2*cos(theta5 - theta7)*(M2 + R2*sin(theta5 - theta7)) + 2*Iyy11*R2*n1^2*sin(theta5 - theta7)*(M1 - R2*cos(theta5 - theta7)) + 2*Lc15*m15*cos(theta1)*sin(theta5)*(cos(theta1)*(S1 + (sqrt((2))*S4)/2 - L1*cos(theta4) - Lc15*cos(theta5)) - Ls13*sin(theta1)) + 2*Lc15*m15*sin(theta1)*sin(theta5)*(sin(theta1)*(S1 + (sqrt((2))*S4)/2 - L1*cos(theta4) - Lc15*cos(theta5)) + Ls13*cos(theta1)) + (2*Ixx12*R2*sin(theta5 - theta7)*(M1 - R2*cos(theta5 - theta7)))/((M1 - R2*cos(theta5 - theta7))^2 + (M2 + R2*sin(theta5 - theta7))^2) + (2*Izz12*R2*cos(theta5 - theta7)*(M2 + R2*sin(theta5 - theta7)))/((M1 - R2*cos(theta5 - theta7))^2 + (M2 + R2*sin(theta5 - theta7))^2)))/2 - (dq3*((Lc11*Ls11*R2*m11*(M2 + R2*sin(theta5 - theta7))*(M2*cos(theta5 - theta7) + M1*sin(theta5 - theta7)) + Lc11*Ls11*R2^2*m11*cos(theta5 - theta7)*(R2 - M1*cos(theta5 - theta7) + M2*sin(theta5 - theta7)))*n1^3 + Lc15*Ls13*m15*cos(theta5)))/2 + (dq3*n1^3*(Lc11*Ls11*R2*m11*(M2 + R2*sin(theta5 - theta7))*(M2*cos(theta5 - theta7) + M1*sin(theta5 - theta7)) + Lc11*Ls11*R2^2*m11*cos(theta5 - theta7)*(R2 - M1*cos(theta5 - theta7) + M2*sin(theta5 - theta7))))/2 + (Lc15*Ls13*dq3*m15*cos(theta5))/2) - dq3*((dq3*((Iyy12*(((M1 - R2*cos(theta5 - theta7))^2*(2*R2*cos(theta5 - theta7)*(M2 + R2*sin(theta5 - theta7)) + 2*R2*sin(theta5 - theta7)*(M1 - R2*cos(theta5 - theta7))))/((M1 - R2*cos(theta5 - theta7))^2 + (M2 + R2*sin(theta5 - theta7))^2)^2 - (2*R2*sin(theta5 - theta7)*(M1 - R2*cos(theta5 - theta7)))/((M1 - R2*cos(theta5 - theta7))^2 + (M2 + R2*sin(theta5 - theta7))^2))*((R2*sin(theta5 - theta7))/sqrt(((M1 - R2*cos(theta5 - theta7))^2 + (M2 + R2*sin(theta5 - theta7))^2)) - ((M1 - R2*cos(theta5 - theta7))*(2*R2*cos(theta5 - theta7)*(M2 + R2*sin(theta5 - theta7)) + 2*R2*sin(theta5 - theta7)*(M1 - R2*cos(theta5 - theta7))))/(2*((M1 - R2*cos(theta5 - theta7))^2 + (M2 + R2*sin(theta5 - theta7))^2)^(3/2)))^2)/((M1 - R2*cos(theta5 - theta7))^2/((M1 - R2*cos(theta5 - theta7))^2 + (M2 + R2*sin(theta5 - theta7))^2) - 1)^2 + (2*Iyy12*((R2*sin(theta5 - theta7))/sqrt(((M1 - R2*cos(theta5 - theta7))^2 + (M2 + R2*sin(theta5 - theta7))^2)) - ((M1 - R2*cos(theta5 - theta7))*(2*R2*cos(theta5 - theta7)*(M2 + R2*sin(theta5 - theta7)) + 2*R2*sin(theta5 - theta7)*(M1 - R2*cos(theta5 - theta7))))/(2*((M1 - R2*cos(theta5 - theta7))^2 + (M2 + R2*sin(theta5 - theta7))^2)^(3/2)))*((R2*cos(theta5 - theta7))/sqrt(((M1 - R2*cos(theta5 - theta7))^2 + (M2 + R2*sin(theta5 - theta7))^2)) + (3*(M1 - R2*cos(theta5 - theta7))*(2*R2*cos(theta5 - theta7)*(M2 + R2*sin(theta5 - theta7)) + 2*R2*sin(theta5 - theta7)*(M1 - R2*cos(theta5 - theta7)))^2)/(4*((M1 - R2*cos(theta5 - theta7))^2 + (M2 + R2*sin(theta5 - theta7))^2)^(5/2)) - ((M1 - R2*cos(theta5 - theta7))*(2*R2^2*cos(theta5 - theta7)^2 + 2*R2^2*sin(theta5 - theta7)^2 + 2*R2*cos(theta5 - theta7)*(M1 - R2*cos(theta5 - theta7)) - 2*R2*sin(theta5 - theta7)*(M2 + R2*sin(theta5 - theta7))))/(2*((M1 - R2*cos(theta5 - theta7))^2 + (M2 + R2*sin(theta5 - theta7))^2)^(3/2)) - (R2*sin(theta5 - theta7)*(2*R2*cos(theta5 - theta7)*(M2 + R2*sin(theta5 - theta7)) + 2*R2*sin(theta5 - theta7)*(M1 - R2*cos(theta5 - theta7))))/((M1 - R2*cos(theta5 - theta7))^2 + (M2 + R2*sin(theta5 - theta7))^2)^(3/2)))/((M1 - R2*cos(theta5 - theta7))^2/((M1 - R2*cos(theta5 - theta7))^2 + (M2 + R2*sin(theta5 - theta7))^2) - 1) - 2*Izz11*R2^2*n1^4*(M2*cos(theta5 - theta7) + M1*sin(theta5 - theta7))*(R2 - M1*cos(theta5 - theta7) + M2*sin(theta5 - theta7))))/2 - (dq3*n1^6*(2*Lc11^2*R2^2*m11*(M1 - R2*cos(theta5 - theta7))^2*(M2*cos(theta5 - theta7) + M1*sin(theta5 - theta7))*(R2 - M1*cos(theta5 - theta7) + M2*sin(theta5 - theta7)) + 2*Lc11^2*R2^3*m11*sin(theta5 - theta7)*(M1 - R2*cos(theta5 - theta7))*(R2 - M1*cos(theta5 - theta7) + M2*sin(theta5 - theta7))^2 + 2*Lc11^2*R2^2*m11*cos(theta1)^2*(M2 + R2*sin(theta5 - theta7))^2*(M2*cos(theta5 - theta7) + M1*sin(theta5 - theta7))*(R2 - M1*cos(theta5 - theta7) + M2*sin(theta5 - theta7)) + 2*Lc11^2*R2^2*m11*sin(theta1)^2*(M2 + R2*sin(theta5 - theta7))^2*(M2*cos(theta5 - theta7) + M1*sin(theta5 - theta7))*(R2 - M1*cos(theta5 - theta7) + M2*sin(theta5 - theta7)) + 2*Lc11^2*R2^3*m11*cos(theta5 - theta7)*cos(theta1)^2*(M2 + R2*sin(theta5 - theta7))*(R2 - M1*cos(theta5 - theta7) + M2*sin(theta5 - theta7))^2 + 2*Lc11^2*R2^3*m11*cos(theta5 - theta7)*sin(theta1)^2*(M2 + R2*sin(theta5 - theta7))*(R2 - M1*cos(theta5 - theta7) + M2*sin(theta5 - theta7))^2))/2)];

G_dot=[(0); - g*m6*(R1*cos(theta4 - theta6) - (R1*sin(theta4 - theta6)*(K2 - R1*cos(theta4 - theta6)))/sqrt(L7^2 - (K2 - R1*cos(theta4 - theta6))^2)) - g*m1*(LC1*cos(theta4) + LC1y*sin(theta4)) - g*m8*(R1*cos(theta4 - theta6) - (R1*sin(theta4 - theta6)*(K2 - R1*cos(theta4 - theta6)))/(2*L8*sqrt(1 - (K2 - R1*cos(theta4 - theta6))^2/L8^2))) - L1*g*cos(theta4)*m10 - L1*g*m3*cos(theta4) - (L1*g*m4*cos(theta4))/2 - L1*g*m14*cos(theta4) - L1*g*m15*cos(theta4) - Lc13*g*m13*cos(theta4) - (R1*g*m7*cos(theta4 - theta6))/2; g*m11*((Lc11*(M2 + R2*sin(theta5 - theta7))*(2*R2*cos(theta5 - theta7)*(M2 + R2*sin(theta5 - theta7)) + 2*R2*sin(theta5 - theta7)*(M1 - R2*cos(theta5 - theta7))))/(2*((M1 - R2*cos(theta5 - theta7))^2 + (M2 + R2*sin(theta5 - theta7))^2)^(3/2)) - (Lc11*R2*cos(theta5 - theta7))/sqrt(((M1 - R2*cos(theta5 - theta7))^2 + (M2 + R2*sin(theta5 - theta7))^2))) + g*m2*(LC2*cos(theta5) - LC2y*sin(theta5)) - L3*g*cos(theta5)*m10 + L2*g*m4*cos(theta5) - LC3*g*m3*cos(theta5) - Lc15*g*m15*cos(theta5) - R2*g*m12*cos(theta5 - theta7)];
tau0=(Mm*d2q+V2+G_dot)*10^-6;

jacobian=[-sin(theta1)*(L1*cos(theta4)+L3*cos(theta5)-S1) -L1*cos(theta1)*sin(theta4) -L3*cos(theta1)*sin(theta5) ;
    cos(theta1)*(L1*cos(theta4)+L3*cos(theta5)-S1) -L1*sin(theta1)*sin(theta4) -L3*sin(theta1)*sin(theta5) ;
    0 L1*cos(theta4) L3*cos(theta5) ];
G_load=[0,0,mload*g].';Fa_load=mload*a;
tau=tau0-jacobian.'*(-Fa_load+G_load)*10^(-6);

adaptive_rate=Mm*(diag(Wn)).'*(diag(Wn))*Z2;%少了10^(-6)？

== matlab function new_inkine_2020/Accelerated ve ==
  data: a input; d2q output; q input; dq input
function d2q  =  accelerated(a,q,dq)
theta1=q(1);theta4=q(2);theta5=q(3);
coder.extrinsic('evalin');
L1=0;L3=0;S1=0;
L1=evalin('base','L1');L3=evalin('base','L3');S1=evalin('base','S1');
% S1=82;L1=600;L3=550;
jacobian=[-sin(theta1)*(L1*cos(theta4)+L3*cos(theta5)-S1) -L1*cos(theta1)*sin(theta4) -L3*cos(theta1)*sin(theta5) ;
    cos(theta1)*(L1*cos(theta4)+L3*cos(theta5)-S1) -L1*sin(theta1)*sin(theta4) -L3*sin(theta1)*sin(theta5) ;
    0 L1*cos(theta4) L3*cos(theta5) ];
H=zeros(3,3,3);
%第一页：J对theta1求偏导
H(:,:,1)=[-cos(theta1)*(L1*cos(theta4) - S1 + L3*cos(theta5)), L1*sin(theta1)*sin(theta4), L3*sin(theta1)*sin(theta5);
    -sin(theta1)*(L1*cos(theta4) - S1 + L3*cos(theta5)), -L1*cos(theta1)*sin(theta4), -L3*cos(theta1)*sin(theta5);
    0,0,0];
%第二页：J对theta4求偏导
H(:,:,2)=[L1*sin(theta1)*sin(theta4), -L1*cos(theta1)*cos(theta4),0;
    -L1*cos(theta1)*sin(theta4), -L1*cos(theta4)*sin(theta1), 0;
    0, -L1*sin(theta4), 0];
%第三页：J对theta5求偏导
H(:,:,3)=[L3*sin(theta1)*sin(theta5), 0, -L3*cos(theta1)*cos(theta5);
    -L3*cos(theta1)*sin(theta5), 0, -L3*cos(theta5)*sin(theta1);
    0,0, -L3*sin(theta5)];
J_dot=dq(1)*H(:,:,1)+dq(2)*H(:,:,2)+dq(3)*H(:,:,3);%笑哭，dq1居然也要变号
d2q =inv(jacobian)*(a-J_dot*dq);%变号后居然吻合了，证明雅克比需要变一次号
% d2q1=d2q(1); 
% 
% n=sqrt((M1 - R2*cos(theta3))^2 + (M2 - R2*sin(theta3))^2);
% phi1=asin((K1-R1*sin(theta2))/Le);
% phi2=acos((K2-R1*cos(theta2))/Le);
% 
% %新的局部雅克比
% J1=-R1*sin(theta2)-R1*cos(theta2)*tan(phi1);
% J2=R1*cos(theta2)+R1*sin(theta2)/tan(phi2);
% J3=(R2*(M2*cos(theta3) - M1*sin(theta3)))/n;
% J1_dot=-dq(2)*((R1^2*cos(theta2)^2)/(Le*sqrt(1 - (K1 - R1*sin(theta2))^2/Le^2)) - R1*cos(theta2) + (R1^2*cos(theta2)^2*(K1 - R1*sin(theta2))^2)/(Le^3*(1 - (K1 - R1*sin(theta2))^2/Le^2)^(3/2)) + (R1*sin(theta2)*(K1 - R1*sin(theta2)))/(Le*sqrt(1 - (K1 - R1*sin(theta2))^2/Le^2)));
% J2_dot=-dq(2)*((R1^2*sin(theta2)^2)/(Le*sqrt(1 - (K2 - R1*cos(theta2))^2/Le^2)) - R1*sin(theta2) + (R1*cos(theta2)*(K2 - R1*cos(theta2)))/(Le*sqrt(1 - (K2 - R1*cos(theta2))^2/Le^2)) + (R1^2*sin(theta2)^2*(K2 - R1*cos(theta2))^2)/(Le^3*(1 - (K2 - R1*cos(theta2))^2/Le^2)^(3/2)));
% J3_dot=-dq(3)*(- (R2*(M1*cos(theta3) + M2*sin(theta3)))/sqrt((M1 - R2*cos(theta3))^2 + (M2 - R2*sin(theta3))^2) - (R2*(M2*cos(theta3) - M1*sin(theta3))*(2*R2*sin(theta3)*(M1 - R2*cos(theta3)) - 2*R2*cos(theta3)*(M2 - R2*sin(theta3))))/(2*((M1 - R2*cos(theta3))^2 + (M2 - R2*sin(theta3))^2)^(3/2)));
% d2t=[0 0 0];
% %二型运动学雅克比求导-线性驱动加速度
% d2t(1)=J1*d2q(2)+J1_dot*dq(2);
% d2t(2)=J2*d2q(2)+J2_dot*dq(2);
% d2t(3)=J3*d2q(3)+J3_dot*dq(3);
